simulink model "B747_mpc_ss_du_pert"  (Simulink 7.9)
settings: Solver=ode4  SolverMode=SingleTasking  StartTime=0.0  StopTime=20  FixedStep=0.001  RelTol=1e-3
values from neighbouring files (symbols this model uses):
  Ac = [0  wr 0 ... (first row only)    [mpc_ss_du_mimo.m]
  Bc = -eye(3)    [mpc_ss_du_mimo.m]
  C = eye(3)    [mpc_ss_du_mimo.m]
  T = 0.005    [mpc_ss_du_mimo.m]
undefined symbols (not defined in the file or in its folder): A, B, KMPC, Phi
settings Model: Creator=Kawakami  LastModifiedBy=Kawakami
settings DataIOCC: SignalLoggingName=sigsOut
settings OptimizationCC: BooleanDataType=off
settings DebuggingCC: SaveWithParameterizedLinksMsg=none  SignalResolutionControl=TryResolveAllWithWarning  SolverPrmCheckMsg=none  MultiTaskDSMMsg=warning  MultiTaskCondExecSysMsg=none  FcnCallInpInsideContextMsg=Use local settings  StrictBusMsg=None
settings HardwareCC: TargetUnknown=on
settings RTWCC: IncludeERTFirstTime=on
settings GRTTargetCC: CombineOutputUpdateFcns=off  GRTInterface=on

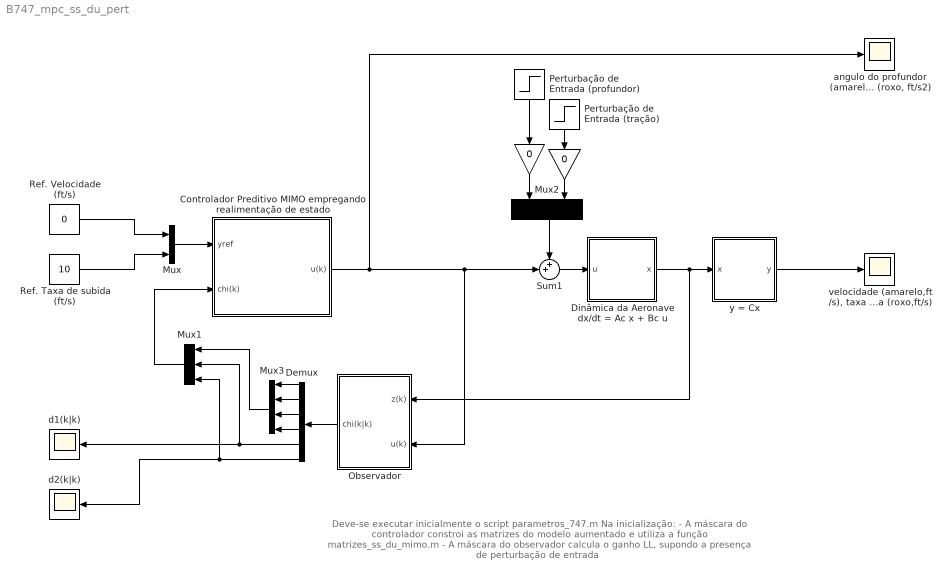
== system B747_mpc_ss_du_pert ==
  note: Deve-se executar inicialmente o script parametros_747.m
      |
      | Na inicialização:
      | - A máscara do controlador constroi as matrizes do modelo aumentado e utiliza a função matrizes_ss_du_mimo.m
      | - A máscara do observador calcula o ganho LL, supondo a presença de perturbação de entrada
  " " : Gain  Gain=0
  "  " : Gain  Gain=0
  Controlador Preditivo MIMO empregando realimentação de estado : Subsystem  mask{rho=[1;1], mu=[1;1], N=10, M=5, A=A, B=B, C=C, T=T}
      mask prompts: rho "Pesos dos controles rho (p x 1)"; mu "Pesos das saídas mu (q x 1)"; N "Horizonte de Predição (N)"; M "Horizonte de Controle (M)"; A "Matriz A (n x n)"; B "Matriz B (n x p)"; C "Matriz C (q x n)"; T "Periodo de amostragem"
      mask init:
      | nold = size(A,1);
      | pold = size(B,2);
      | qold = size(C,1);
      | Ab = [A B ; zeros(pold,nold) eye(pold)];
      | Bb = [B;zeros(pold,pold)];
      | Cb = [C zeros(qold,pold)];
      | 
      | [KMPC,Phi] = matrizes_ss_du_mimo(Ab,Bb,Cb,N,M,mu,rho);
      | n = size(Ab,1);
      | p = size(Bb,2);
      | q = size(Cb,1);
  Demux : Demux  Outputs=6
  Dinâmica da Aeronave dx/dt = Ac x + Bc u : Subsystem
  Mux : Mux  Inputs=2
  Mux1 : Mux  Inputs=3
  Mux2 : Mux  Inputs=2
  Mux3 : Mux
  Observador : Subsystem  mask{A=A, B=B, Cz=eye(4), T=T, poles=[0.5,0.51,0.52,0.53,0.54,0.55]}
      mask prompts: A "Matriz A"; B "Matriz B"; Cz "Matriz Cz"; T "Periodo de amostragem"; poles "Pólos para a dinâmica do erro de estimacao"
      mask init:
      | n = size(A,1);
      | p = size(B,2);
      | nz = size(Cz,1);
      | Ab = [A B ; zeros(p,n) eye(p)];
      | Bb = [B;zeros(p,p)];
      | Czb = [Cz zeros(nz,p)];
      | L = place(Ab',Czb',poles)';
      | LL = inv(Ab)*L;
  Perturbação de Entrada (profundor) : Step  Time=4  After=2  SampleTime=0
  Perturbação de Entrada (tração) : Step  Time=8  After=2  SampleTime=0
  Ref. Taxa de subida (ft/s) : Constant  Value=10
  Ref. Velocidade (ft/s) : Constant  Value=0
  Sum1 : Sum  Inputs=++|  SaturateOnIntegerOverflow=on
  "angulo do profundor (amarelo, crad) tração específica (roxo, ft/s2)" : Scope
      settings: TimeRange=10  YMin=-6  YMax=3  SaveName=y1
  d1(k|k) : Scope
      settings: TimeRange=10  YMin=-0.5  YMax=2  SaveName=y2
  d2(k|k) : Scope
      settings: TimeRange=10  YMin=-0.5  YMax=2  SaveName=y3
  "velocidade (amarelo,ft/s), taxa de subida (roxo,ft/s)" : Scope
      settings: TimeRange=10  YMin=-2  YMax=12  SaveName=y
  y = Cx : Subsystem
  wires:
  Controlador Preditivo MIMO empregando realimentação de estado/1(u(k)) -> "angulo do profundor (amarelo, crad) tração específica (roxo, ft/s2)"/1, Sum1/2, Observador/2(u(k))
  Dinâmica da Aeronave dx/dt = Ac x + Bc u/1(x) -> y = Cx/1(x), Observador/1(z(k))
  Mux/1 -> Controlador Preditivo MIMO empregando realimentação de estado/1(yref)
  Ref. Velocidade (ft/s)/1 -> Mux/1
  Ref. Taxa de subida (ft/s)/1 -> Mux/2
  Sum1/1 -> Dinâmica da Aeronave dx/dt = Ac x + Bc u/1(u)
  y = Cx/1(y) -> "velocidade (amarelo,ft/s), taxa de subida (roxo,ft/s)"/1
  Demux/5 -> Mux1/2, d1(k|k)/1
  Demux/6 -> Mux1/3, d2(k|k)/1
  Observador/1(chi(k|k)) -> Demux/1
  Mux1/1 -> Controlador Preditivo MIMO empregando realimentação de estado/2(chi(k))
  Demux/1 -> Mux3/1
  Demux/2 -> Mux3/2
  Demux/3 -> Mux3/3
  Demux/4 -> Mux3/4
  Mux3/1 -> Mux1/1
  Perturbação de Entrada (profundor)/1 -> "  "/1
  Perturbação de Entrada (tração)/1 -> " "/1
  "  "/1 -> Mux2/1
  " "/1 -> Mux2/2
  Mux2/1 -> Sum1/1

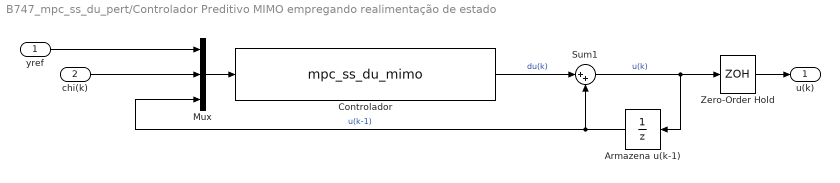
== system B747_mpc_ss_du_pert/Controlador Preditivo MIMO empregando realimentação de estado ==
  yref : Inport
  chi(k) : Inport  Port=2
  Armazena u(k-1) : UnitDelay  SampleTime=T
  Controlador : S-Function  FunctionName=mpc_ss_du_mimo  Parameters=KMPC,Phi,p,q,n,N,T  EnableBusSupport=off
  Mux : Mux  Inputs=3
  Sum1 : Sum  Inputs=|++  SaturateOnIntegerOverflow=on  InputSameDT=on  OutDataTypeStr=Inherit: Same as first input
  Zero-Order Hold : ZeroOrderHold  SampleTime=T
  u(k) : Outport
  wires:
  Mux/1 -> Controlador/1
  Zero-Order Hold/1 -> u(k)/1
  chi(k)/1 -> Mux/2
  yref/1 -> Mux/1
  Sum1/1 -> Zero-Order Hold/1, Armazena u(k-1)/1  "u(k)"
  Armazena u(k-1)/1 -> Sum1/2, Mux/3  "u(k-1)"
  Controlador/1 -> Sum1/1  "du(k)"

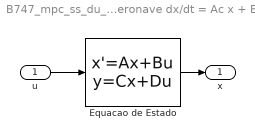
== system B747_mpc_ss_du_pert/Dinâmica da Aeronave dx/dt = Ac x + Bc u ==
  u : Inport
  Equacao de Estado : StateSpace  A=Ac  B=Bc  C=eye(size(A,1),size(A,1))  D=zeros(size(A,1),size(B,2))  X0=zeros(size(A,1),1)
  x : Outport
  wires:
  u/1 -> Equacao de Estado/1
  Equacao de Estado/1 -> x/1

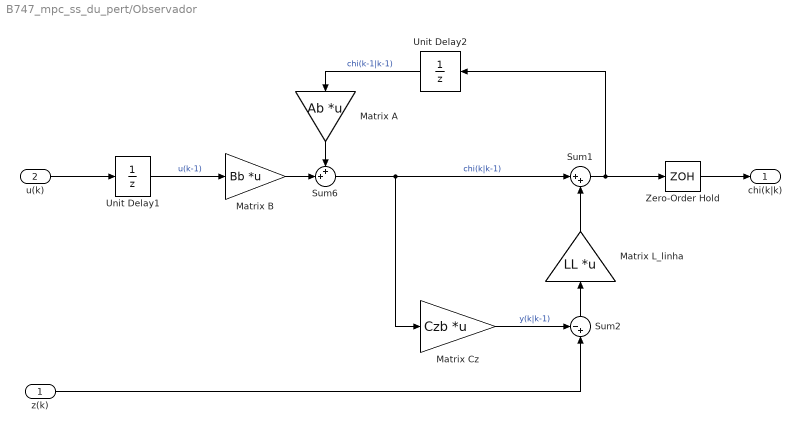
== system B747_mpc_ss_du_pert/Observador ==
  z(k) : Inport
  u(k) : Inport  Port=2
  Matrix L_linha : Gain  Gain=LL  Multiplication=Matrix(K*u)  SaturateOnIntegerOverflow=on  OutDataTypeStr=Inherit: Same as input  ParamDataTypeStr=Inherit: Same as input
  Matrix A : Gain  Gain=Ab  Multiplication=Matrix(K*u)  SaturateOnIntegerOverflow=on  OutDataTypeStr=Inherit: Same as input  ParamDataTypeStr=Inherit: Same as input
  Matrix B : Gain  Gain=Bb  Multiplication=Matrix(K*u)  SaturateOnIntegerOverflow=on  OutDataTypeStr=Inherit: Same as input  ParamDataTypeStr=Inherit: Same as input
  Matrix Cz : Gain  Gain=Czb  Multiplication=Matrix(K*u)  SaturateOnIntegerOverflow=on  OutDataTypeStr=Inherit: Same as input  ParamDataTypeStr=Inherit: Same as input
  Sum1 : Sum  Inputs=|++  SaturateOnIntegerOverflow=on
  Sum2 : Sum  Inputs=-+|  SaturateOnIntegerOverflow=on
  Sum6 : Sum  Inputs=++|  SaturateOnIntegerOverflow=on
  Unit Delay1 : UnitDelay  SampleTime=T
  Unit Delay2 : UnitDelay  SampleTime=T
  Zero-Order Hold : ZeroOrderHold  SampleTime=T
  chi(k|k) : Outport
  wires:
  u(k)/1 -> Unit Delay1/1
  Unit Delay1/1 -> Matrix B/1  "u(k-1)"
  Matrix B/1 -> Sum6/2
  Sum6/1 -> Sum1/1, Matrix Cz/1  "chi(k|k-1)"
  Sum1/1 -> Unit Delay2/1, Zero-Order Hold/1
  Matrix A/1 -> Sum6/1
  Unit Delay2/1 -> Matrix A/1  "chi(k-1|k-1)"
  Matrix L_linha/1 -> Sum1/2
  Sum2/1 -> Matrix L_linha/1
  Matrix Cz/1 -> Sum2/1  "y(k|k-1)"
  z(k)/1 -> Sum2/2
  Zero-Order Hold/1 -> chi(k|k)/1

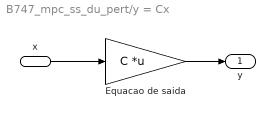
== system B747_mpc_ss_du_pert/y = Cx ==
  x : Inport
  Equacao de saida : Gain  Gain=C  Multiplication=Matrix(K*u)  SaturateOnIntegerOverflow=on  OutDataTypeStr=Inherit: Same as input  ParamDataTypeStr=Inherit: Same as input
  y : Outport
  wires:
  x/1 -> Equacao de saida/1
  Equacao de saida/1 -> y/1
